simulink model "ADRC_2_MODEL"  (Simulink 7.6)
settings: Solver=ode45  StartTime=0.0  StopTime=200  RelTol=1e-3
settings Model: Creator=Administrator  LastModifiedBy=Administrator
settings DebuggingCC: AlgebraicLoopMsg=none  ArtificialAlgebraicLoopMsg=none  SolverPrmCheckMsg=none  UnknownTsInhSupMsg=none

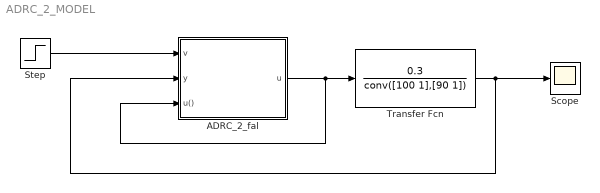
== system ADRC_2_MODEL ==
  ADRC_2_fal : Subsystem  AncestorBlock=ADRC/ADRC/ADRC_2rd/ADRC_2_fal  mask{r=0.01, h=0.1, B01=100, B02=300, B03=1000, D=0.1, b=1, k1=10, k2=5, Ds=0.1}
      mask prompts: B01 "B01="; B02 "B02="; B03 "B03="; D "D="; k1 "k1="; k2 "k2="; Ds "Ds="
  Scope : Scope
  Step : Step  SampleTime=0
  Transfer Fcn : TransferFcn  Numerator=0.3  Denominator=conv([100 1],[90 1])
  wires:
  Step/1 -> ADRC_2_fal/1(v)
  ADRC_2_fal/1(u) -> Transfer Fcn/1, ADRC_2_fal/3(u())
  Transfer Fcn/1 -> Scope/1, ADRC_2_fal/2(y)

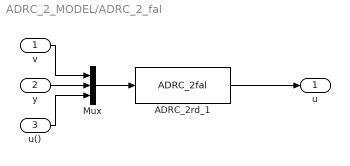
== system ADRC_2_MODEL/ADRC_2_fal ==
  v : Inport
  y : Inport  Port=2
  u() : Inport  Port=3
  ADRC_2rd_1 : S-Function  FunctionName=ADRC_2fal  Parameters=r,h,B01,B02,B03,D,b,k1,k2,Ds  EnableBusSupport=off  mask{r=0, h=0, B01=0, B02=0, B03=0, D=0, b=0, k1=0, k2=0, Ds=0}
      mask prompts: r "r="; h "h="; B01 "B01="; B02 "B02="; B03 "B03="
  Mux : Mux  Inputs=3
  u : Outport
  wires:
  ADRC_2rd_1/1 -> u/1
  v/1 -> Mux/1
  y/1 -> Mux/2
  Mux/1 -> ADRC_2rd_1/1
  u()/1 -> Mux/3
